simulink model "AZ5forceCntrl"  (R2016b)
settings: Solver=FixedStepAuto  StartTime=0.0  StopTime=55  RelTol=1e-3
libraries: Rayannik x3, simulink x1
settings Model: ExtModeTrigDuration=1000001  Creator=user  LastModifiedBy=Alireza7
settings DataIOCC: LimitDataPoints=on  SaveFormat=Array
settings OptimizationCC: BlockReduction=off  BooleanDataType=off
settings DebuggingCC: SaveWithParameterizedLinksMsg=none  UnderspecifiedInitializationDetection=Classic  MergeDetectMultiDrivingBlocksExec=none  SignalResolutionControl=TryResolveAllWithWarning  SFUnexpectedBacktrackingDiag=warning  SFNoUnconditionalDefaultTransitionDiag=warning  SFExecutionAtInitializationDiag=none
settings ModelReferenceCC: PropagateSignalLabelsOutOfModel=off
settings RTWCC: SystemTargetFile=sldrt.tlc  TemplateMakefile=sldrt.tmf  Description=Simulink Desktop Real-Time  RTWCompilerOptimization=on
settings CodeAppCC: MaxIdLength=95
settings SimulinkDesktopRealTimeCC: TargetPreCompLibLocation=C:\Program Files\MATLAB\R2016b\toolbox\sldrt\lib\win64  TargetLangStandard=C89/C90 (ANSI)  SupportVariableSizeSignals=off
settings ConfigComp: CovMetricSettings=dw  CovHtmlReporting=on  CovSaveCumulativeToWorkspaceVar=on  CovSaveSingleToWorkspaceVar=on  CovExternalEMLEnable=off  CovSFcnEnable=off

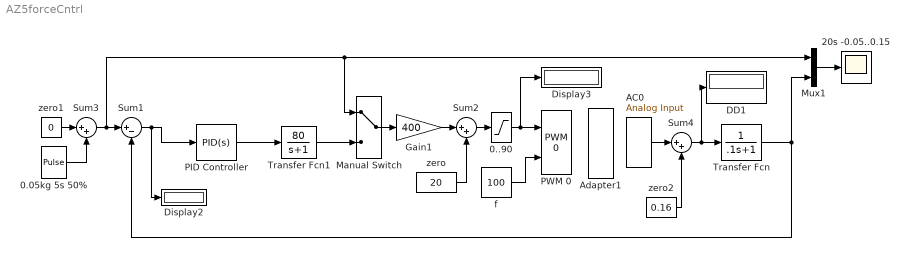
== system AZ5forceCntrl ==
  0..90 : Saturate  UpperLimit=90  LowerLimit=0
  0.05kg 5s 50% : DiscretePulseGenerator  PulseType=Time based  Amplitude=0.1  Period=10  PulseWidth=50
  20s -0.05..0.15 : Scope
  AC0 : Rayannik/Analog Input  Priority=2  CH=0  vr=2.5  ou=Analog  inrr=-10 ~ +10
  Adapter1 : Rayannik/Adapter  SystemSampleTime=-1
      link override Packet Input1: SampleTime=Ts  MaxMissedTicks=1000000  ShowMissedTicks=off  YieldWhenWaiting=off  DrvName=Standard_Devices/Serial_Port  DrvAddress=3  DrvOptions=[9600 8 0 0 0 0 0 0]  PacketSize=33  DataTypes='33*uint8'  ShowReady=off  ShowError=off  PacketID=1  ByteOrder=1  ShowTimestamp=off
      link override Packet Output1: SampleTime=Ts  MaxMissedTicks=10000000  ShowMissedTicks=off  YieldWhenWaiting=off  DrvName=Standard_Devices/Serial_Port  DrvAddress=3  DrvOptions=[9600 8 0 0 0 0 0 0]  PacketSize=31  DataTypes='31*uint8'  ShowReady=off  ShowError=off  PacketID=1  ByteOrder=1  InitialValue=[]  FinalValue=[]
  DD1 : Display
  Display2 : Display
  Display3 : Display
  Gain1 : Gain  Gain=400
  Manual Switch : ManualSwitch
  Mux1 : Mux  Inputs=2
  PID Controller : simulink/Continuous/PID Controller  Controller=PID  TimeDomain=Continuous-time  SampleTime=-1  IntegratorMethod=Forward Euler  FilterMethod=Forward Euler  Form=Parallel  UseFilter=on  ControllerParametersSource=internal  P=80  I=1  D=0  N=100  InitialConditionSource=internal  InitialConditionForIntegrator=0  InitialConditionForFilter=0  ExternalReset=none  LimitOutput=off  UpperSaturationLimit=inf  LowerSaturationLimit=-inf  LinearizeAsGain=on  AntiWindupMode=none  Kb=1  TrackingMode=off  Kt=1  PParamMin=[]  PParamMax=[]  IParamMin=[]  IParamMax=[]  DParamMin=[]  DParamMax=[]  NParamMin=[]  NParamMax=[]  KbParamMin=[]  KbParamMax=[]  KtParamMin=[]  KtParamMax=[]  POutMin=[]  POutMax=[]  IOutMin=[]  IOutMax=[]  DOutMin=[]  DOutMax=[]  NOutMin=[]  NOutMax=[]  KbOutMin=[]  KbOutMax=[]  KtOutMin=[]  KtOutMax=[]  IntegratorOutMin=[]  IntegratorOutMax=[]  FilterOutMin=[]  FilterOutMax=[]  SumOutMin=[]  SumOutMax=[]  SumI1OutMin=[]  SumI1OutMax=[]  SumI2OutMin=[]  SumI2OutMax=[]  SumI3OutMin=[]  SumI3OutMax=[]  SumDOutMin=[]  SumDOutMax=[]  SaturationOutMin=[]  SaturationOutMax=[]  IntegratorContinuousStateAttributes=''  IntegratorStateMustResolveToSignalObject=off  IntegratorRTWStateStorageClass=Auto  FilterContinuousStateAttributes=''  FilterStateMustResolveToSignalObject=off  FilterRTWStateStorageClass=Auto  DifferentiatorICPrevScaledInput=0  DifferentiatorOutMin=[]  DifferentiatorOutMax=[]
  PWM 0 : Rayannik/PWM 0  Priority=2  md=Constant Frequency Mode
  Sum1 : Sum  Inputs=|+-
  Sum2 : Sum  Inputs=|++
  Sum3 : Sum  Inputs=|++
  Sum4 : Sum  Inputs=|++
  Transfer Fcn : TransferFcn  Denominator=[.1 1]
  Transfer Fcn1 : TransferFcn  Numerator=[80]  Denominator=[1 1]
  f : Constant  Value=100
  zero : Constant  Value=20  SampleTime=1
  zero1 : Constant  Value=0  SampleTime=1
  zero2 : Constant  Value=0.16  SampleTime=1
  wires:
  Sum3/1 -> Manual Switch/1, Mux1/1, Sum1/1
  Mux1/1 -> 20s -0.05..0.15/1
  Sum4/1 -> Transfer Fcn/1, DD1/1
  0..90/1 -> Display3/1, PWM 0/1
  Sum2/1 -> 0..90/1
  f/1 -> PWM 0/2
  zero/1 -> Sum2/2
  Transfer Fcn/1 -> Mux1/2, Sum1/2
  0.05kg 5s 50%/1 -> Sum3/2
  zero1/1 -> Sum3/1
  Manual Switch/1 -> Gain1/1
  AC0/1 -> Sum4/1
  zero2/1 -> Sum4/2
  Gain1/1 -> Sum2/1
  Transfer Fcn1/1 -> Manual Switch/2
  Sum1/1 -> PID Controller/1, Display2/1
  PID Controller/1 -> Transfer Fcn1/1
